simulink model "Turntable_Spawn"  (R2021a)
settings: Solver=ode4  StartTime=0.0  StopTime=inf  FixedStep=1/120  RelTol=1e-3  EnableMultiTasking=on
libraries: quarc_library x9, simulink x2
settings Model: SimulationMode=external  ExtModeTrigDuration=10000  Creator=MLevis  LastModifiedBy=swhitmell
settings SolverCC: AlgebraicLoopSolver=TrustRegion  PositivePriorityOrder=on
settings DataIOCC: ReturnWorkspaceOutputs=off
settings DebuggingCC: SFMachineParentedDataDiag=warning  ArithmeticOperatorsInVariantConditions=warning
settings HardwareCC: ProdBitPerPointer=32  ProdBitPerSizeT=32  ProdBitPerPtrDiffT=32  ProdLargestAtomicInteger=Long  ProdLargestAtomicFloat=Double  ProdWordSize=32  ProdHWDeviceType=ARM Compatible->ARM Cortex
settings SFSimCC: SimUseLocalCustomCode=off  CustomCodeUndefinedFunction=UseInterfaceOnly
settings RTWCC: Description=QUARC Linux Raspberry Pi 3 Target (QBot 2e) Using Toolchain  SystemTargetFile=quarc_linux_pi_3.tlc  TemplateMakefile=quarc_default_tmf  RTWUseLocalCustomCode=off  Toolchain=QUARC linux_pi_3 | gmake (64-bit Windows)  BuildConfiguration=Faster Runs
settings CodeAppCC: StateflowObjectComments=on
settings STFCustomTargetCC: TargetLangStandard=C99 (ISO)  ConcurrentExecutionCompliant=on  SystemTargetFile=quarc_linux_pi_3.tlc
settings GRTTargetCC: ParMdlRefBuildCompliant=off  CompOptLevelCompliant=off  CombineOutputUpdateFcns=off  MatFileLogging=off  CPPClassGenCompliant=off  GRTInterface=on  ExtMode=on  ExtModeMexFile=quarc_comm  ExtModeMexArgs='-w -d /tmp -uri %u'
settings ConfigComp: CovMetricSettings=dswe

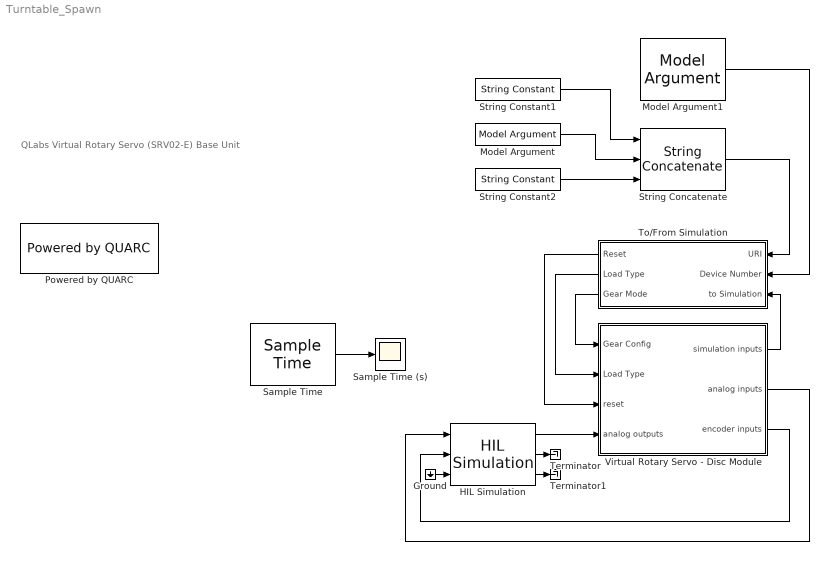
== system Turntable_Spawn ==
  note: QLabs Virtual Rotary Servo (SRV02-E)
      | Base Unit
  Ground : Ground
  HIL Simulation : quarc_library/Data Acquisition/Generic/Configuration/HIL Simulation  uri=tcpip://localhost:18940  board_type=q8_usb  board_id=0  sample_time=qc_get_step_size  active=on  num_clocks=1  num_interrupts=0  num_analog_inputs=8  num_analog_outputs=8  initial_analog=[]  num_digital_io=0  num_digital_inputs=8  num_digital_outputs=8  initial_digital=[]  num_encoder_inputs=8  num_pwm_outputs=8  initial_pwm=[]  other_inputs=[]  other_outputs=[]  initial_other=[]  integer_properties=[]  double_properties=[]  string_properties=[]
      settings: SourceProductName=QUARC Targets
  Model Argument : quarc_library/Sources/Signals/Model Argument  argument_name=hostname  has_value=on  data_type_mode=Specify via dialog  data_type=char  max_length=80  default_value=0  default_string=localhost  variable_size=off
      settings: AttributesFormatString=(-%<argument_name>)  SourceProductName=QUARC Targets
  Model Argument1 : quarc_library/Sources/Signals/Model Argument  argument_name=devicenum  has_value=on  data_type_mode=Specify via dialog  data_type=int32  max_length=80  default_value=0  variable_size=off
      settings: AttributesFormatString=(-%<argument_name>)  SourceProductName=QUARC Targets
  Powered by QUARC : quarc_library/Logos/Powered by QUARC
  Sample Time : quarc_library/Sources/Time/Sample Time  Priority=-99  sample_time=qc_get_step_size
  Sample Time (s) : Scope
  String Concatenate : quarc_library/Strings/String Concatenate  num_inputs=3  max_length=80  output_size=Inherit from input
      settings: SourceProductName=QUARC Targets
  String Constant1 : quarc_library/Strings/String Constant  string_value=tcpip://  evaluate_string=off  string_type=text  max_length=80  sample_time=inf  variable_size=off
      settings: AttributesFormatString="\"tcpip://\""  SourceProductName=QUARC Targets
  String Constant2 : quarc_library/Strings/String Constant  string_value=:18000?nagle='off'  evaluate_string=off  string_type=text  max_length=80  sample_time=inf  variable_size=off
      settings: AttributesFormatString="\":18000?nagle='off'\""  SourceProductName=QUARC Targets
  Terminator : Terminator
  Terminator1 : Terminator
  To/From Simulation : Subsystem
  Virtual Rotary Servo - Disc Module : Subsystem
  wires:
  To/From Simulation/2(Load Type) -> Virtual Rotary Servo - Disc Module/2(Load Type)
  Virtual Rotary Servo - Disc Module/3(encoder inputs) -> HIL Simulation/2
  Virtual Rotary Servo - Disc Module/2(analog inputs) -> HIL Simulation/1
  HIL Simulation/1 -> Virtual Rotary Servo - Disc Module/4(analog outputs)
  Sample Time/1 -> Sample Time (s)/1
  Virtual Rotary Servo - Disc Module/1(simulation inputs) -> To/From Simulation/3(to Simulation)
  To/From Simulation/1(Reset) -> Virtual Rotary Servo - Disc Module/3(reset)
  Ground/1 -> HIL Simulation/3
  HIL Simulation/2 -> Terminator/1
  HIL Simulation/3 -> Terminator1/1
  To/From Simulation/3(Gear Mode) -> Virtual Rotary Servo - Disc Module/1(Gear Config)
  Model Argument/1 -> String Concatenate/2
  String Constant2/1 -> String Concatenate/3
  String Constant1/1 -> String Concatenate/1
  String Concatenate/1 -> To/From Simulation/1(URI)
  Model Argument1/1 -> To/From Simulation/2(Device Number)

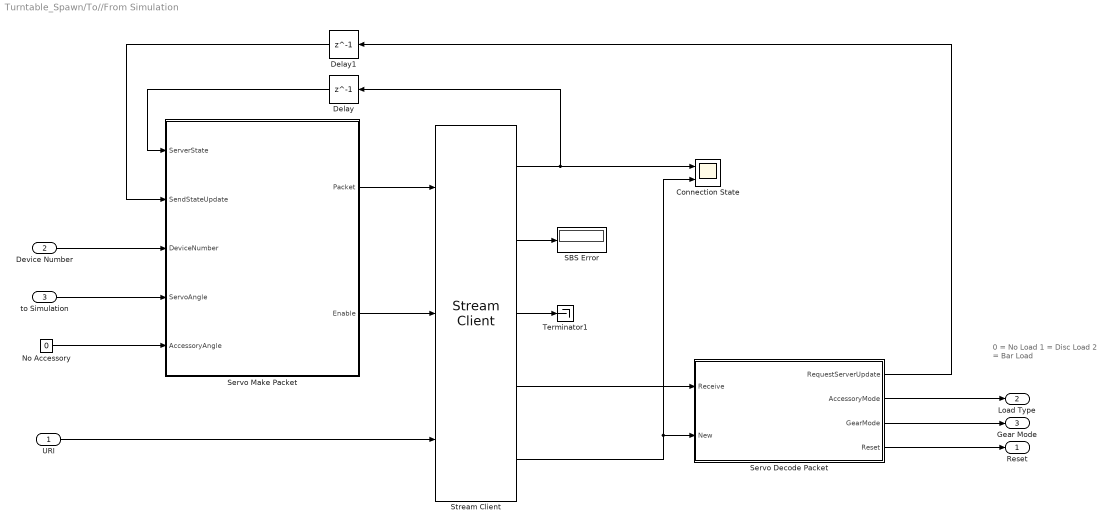
== system Turntable_Spawn/To//From Simulation ==
  note: 0 = No Load
      | 1 = Disc Load
      | 2 = Bar Load
  URI : Inport
  Device Number : Inport  Port=2
  to Simulation : Inport  Port=3
  "Connection State " : Scope  NumInputPorts=2
  Delay : Delay  DelayLength=1
  Delay1 : Delay  DelayLength=1
  No Accessory : Constant  Value=0
  SBS Error : Display
  Servo Decode Packet : MATLAB Function  TreatAsAtomicUnit=on
  Servo Make Packet : MATLAB Function  TreatAsAtomicUnit=on
  Stream Client : quarc_library/Communications/Basic/Stream Client  uri_source=External input port  uri=tcpip://remotehost:18000  apply_uri_to_all_configs=on  send_buffer_size=65537  receive_buffer_size=100000  byte_order=little endian (Intel - LSB first)  optimization=Minimum latency  send_options=Send all data  receive_options=Receive all data  default_value=[0]  sample_time=qc_get_step_size  active=on  implementation=Use blocking I/O in a separate thread  send_fifo_size=3  receive_fifo_size=3  send_priority=0  receive_priority=0  send_dimensions=on  receive_dimensions=on  max_dimensions=100000  data_type=uint8  type_expr=BusObject
  Terminator1 : Terminator
  Reset : Outport  VectorParamsAs1DForOutWhenUnconnected=off
  Load Type : Outport  Port=2  VectorParamsAs1DForOutWhenUnconnected=off
  Gear Mode : Outport  Port=3  VectorParamsAs1DForOutWhenUnconnected=off
  wires:
  Servo Decode Packet/2(AccessoryMode) -> Load Type/1
  Stream Client/2 -> SBS Error/1
  Servo Decode Packet/4(Reset) -> Reset/1
  Stream Client/3 -> Terminator1/1
  Stream Client/1 -> Delay/1, "Connection State "/1
  Servo Make Packet/2(Enable) -> Stream Client/2
  Servo Decode Packet/1(RequestServerUpdate) -> Delay1/1
  Stream Client/5 -> "Connection State "/2, Servo Decode Packet/2(New)
  Servo Make Packet/1(Packet) -> Stream Client/1
  Stream Client/4 -> Servo Decode Packet/1(Receive)
  No Accessory/1 -> Servo Make Packet/5(AccessoryAngle)
  to Simulation/1 -> Servo Make Packet/4(ServoAngle)
  Device Number/1 -> Servo Make Packet/3(DeviceNumber)
  Delay1/1 -> Servo Make Packet/2(SendStateUpdate)
  Delay/1 -> Servo Make Packet/1(ServerState)
  Servo Decode Packet/3(GearMode) -> Gear Mode/1
  URI/1 -> Stream Client/3

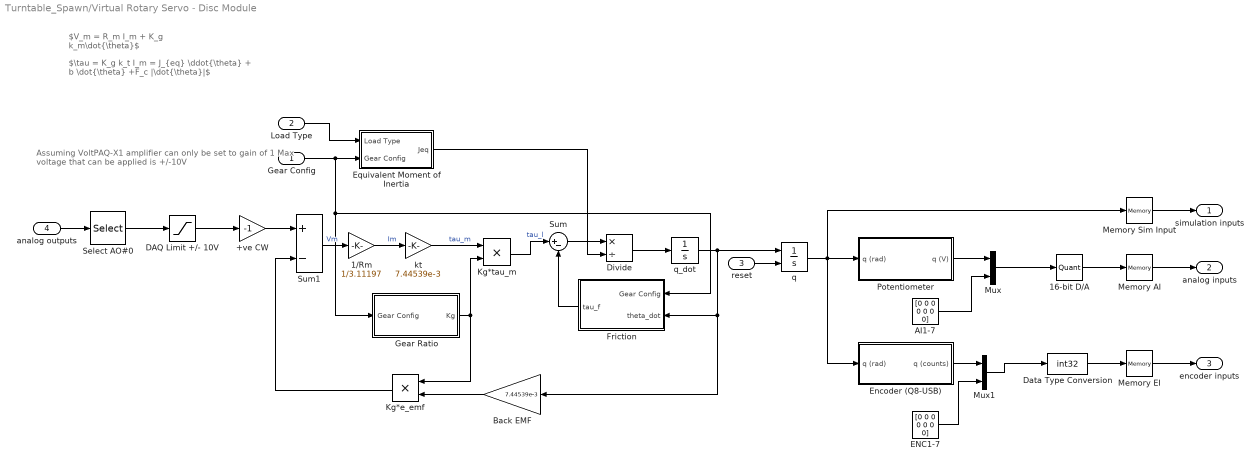
== system Turntable_Spawn/Virtual Rotary Servo - Disc Module ==
  note: $\tau = K_g k_t I_m = J_{eq} \ddot{\theta} + b \dot{\theta} +F_c |\dot{\theta}|$
  note: Assuming VoltPAQ-X1 amplifier can only be set to gain of 1
      | Max voltage that can be applied is +/-10V
  note: $V_m = R_m I_m + K_g k_m\dot{\theta}$
  Gear Config : Inport
  Load Type : Inport  Port=2
  reset : Inport  Port=3
  analog outputs : Inport  Port=4
  +ve CW : Gain  Gain=-1
  1/Rm : Gain  Gain=1/3.11197
  16-bit D/A : Quantizer  QuantizationInterval=1/2^16
  AI1-7 : Constant  Value=[0 0 0 0 0 0 0]
  Back EMF : Gain  Gain=7.44539e-3
  DAQ Limit +/- 10V : Saturate  UpperLimit=10  LowerLimit=-10
  Data Type Conversion : DataTypeConversion  OutDataTypeStr=int32
  Divide : Product  Inputs=*/
  ENC1-7 : Constant  Value=[0 0 0 0 0 0 0]
  Encoder (Q8-USB) : Subsystem
  Equivalent Moment of Inertia : Subsystem
  Friction : Subsystem
  Gear Ratio : Subsystem
  Kg*e_emf : Product
  Kg*tau_m : Product
  Memory AI : Memory  InheritSampleTime=on
  Memory EI : Memory  InheritSampleTime=on
  Memory Sim Input : Memory  InheritSampleTime=on
  Mux : Mux  Inputs=2
  Mux1 : Mux  Inputs=2
  Potentiometer : Subsystem
  Select AO#0 : Selector  InputPortWidth=8  IndexOptions=Index vector (dialog)  Indices=[1]  OutputSizes=1
  Sum : Sum  Inputs=|+-
  Sum1 : Sum  Inputs=+-
  kt : Gain  Gain=7.44539e-3
  q : Integrator  ExternalReset=either
  q_dot : Integrator
  simulation inputs : Outport  VectorParamsAs1DForOutWhenUnconnected=off
  analog inputs : Outport  Port=2  VectorParamsAs1DForOutWhenUnconnected=off
  encoder inputs : Outport  Port=3  VectorParamsAs1DForOutWhenUnconnected=off
  wires:
  kt/1 -> Kg*tau_m/1  "tau_m"
  Mux/1 -> 16-bit D/A/1
  Potentiometer/1(q (V)) -> Mux/1
  AI1-7/1 -> Mux/2
  Mux1/1 -> Data Type Conversion/1
  Encoder (Q8-USB)/1(q (counts)) -> Mux1/1
  ENC1-7/1 -> Mux1/2
  Equivalent Moment of Inertia/1(Jeq) -> Divide/2
  Divide/1 -> q_dot/1
  Sum/1 -> Divide/1
  Friction/1(tau_f) -> Sum/2
  Gear Ratio/1(Kg) -> Kg*e_emf/1, Kg*tau_m/2
  Back EMF/1 -> Kg*e_emf/2
  Gear Config/1 -> Equivalent Moment of Inertia/2(Gear Config), Friction/1(Gear Config), Gear Ratio/1(Gear Config)
  q/1 -> Memory Sim Input/1, Potentiometer/1(q (rad)), Encoder (Q8-USB)/1(q (rad))
  reset/1 -> q/2
  Load Type/1 -> Equivalent Moment of Inertia/1(Load Type)
  16-bit D/A/1 -> Memory AI/1
  +ve CW/1 -> Sum1/1
  Data Type Conversion/1 -> Memory EI/1
  analog outputs/1 -> Select AO#0/1
  Select AO#0/1 -> DAQ Limit +/- 10V/1
  Kg*tau_m/1 -> Sum/1  "tau_l"
  Kg*e_emf/1 -> Sum1/2
  q_dot/1 -> Friction/2(theta_dot), Back EMF/1, q/1
  Sum1/1 -> 1/Rm/1  "Vm"
  1/Rm/1 -> kt/1  "Im"
  DAQ Limit +/- 10V/1 -> +ve CW/1
  Memory AI/1 -> analog inputs/1
  Memory EI/1 -> encoder inputs/1
  Memory Sim Input/1 -> simulation inputs/1

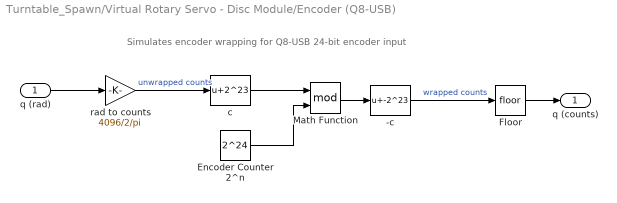
== system Turntable_Spawn/Virtual Rotary Servo - Disc Module/Encoder (Q8-USB) ==
  note: Simulates encoder wrapping for Q8-USB 24-bit encoder input
  q (rad) : Inport
  -c : Bias  Bias=-2^23
  Encoder Counter 2^n : Constant  Value=2^24
  Floor : Rounding
  Math Function : Math  Operator=mod  SignedPower=on  SaturateOnIntegerOverflow=on
  c : Bias  Bias=2^23
  rad to counts : Gain  Gain=4096/2/pi
  q (counts) : Outport  VectorParamsAs1DForOutWhenUnconnected=off
  wires:
  Floor/1 -> q (counts)/1
  -c/1 -> Floor/1  "wrapped counts"
  rad to counts/1 -> c/1  "unwrapped counts"
  Encoder Counter 2^n/1 -> Math Function/2
  c/1 -> Math Function/1
  q (rad)/1 -> rad to counts/1
  Math Function/1 -> -c/1

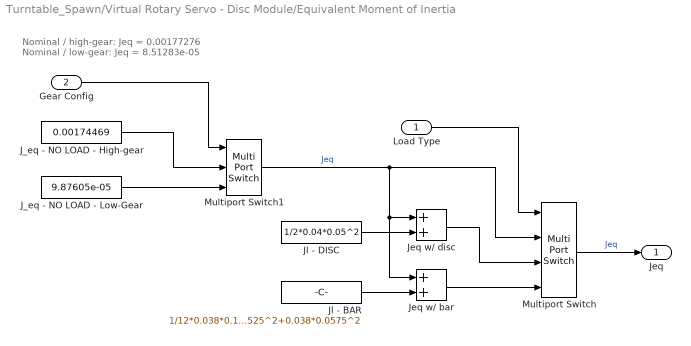
== system Turntable_Spawn/Virtual Rotary Servo - Disc Module/Equivalent Moment of Inertia ==
  note: Nominal / high-gear: Jeq = 0.00177276
      | Nominal / low-gear: Jeq = 8.51283e-05
  Load Type : Inport
  Gear Config : Inport  Port=2
  J_eq - NO LOAD - High-gear : Constant  Value=0.00174469
  J_eq - NO LOAD - Low-Gear : Constant  Value=9.87605e-05
  Jeq w/ bar : Sum
  Jeq w/ disc : Sum
  Jl - BAR : Constant  Value=1/12*0.038*0.1525^2+0.038*0.0575^2
  Jl - DISC : Constant  Value=1/2*0.04*0.05^2
  Multiport Switch : MultiPortSwitch  DataPortOrder=Zero-based contiguous  zeroidx=on
  Multiport Switch1 : MultiPortSwitch  DataPortOrder=Zero-based contiguous  Inputs=2  zeroidx=on
  Jeq : Outport  VectorParamsAs1DForOutWhenUnconnected=off
  wires:
  J_eq - NO LOAD - Low-Gear/1 -> Multiport Switch1/3
  J_eq - NO LOAD - High-gear/1 -> Multiport Switch1/2
  Multiport Switch/1 -> Jeq/1  "Jeq"
  Multiport Switch1/1 -> Multiport Switch/2, Jeq w/ disc/1, Jeq w/ bar/1  "Jeq"
  Gear Config/1 -> Multiport Switch1/1
  Jeq w/ disc/1 -> Multiport Switch/3
  Load Type/1 -> Multiport Switch/1
  Jeq w/ bar/1 -> Multiport Switch/4
  Jl - BAR/1 -> Jeq w/ bar/2
  Jl - DISC/1 -> Jeq w/ disc/2

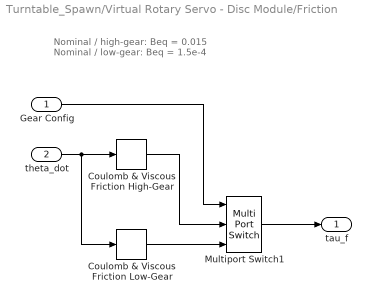
== system Turntable_Spawn/Virtual Rotary Servo - Disc Module/Friction ==
  note: Nominal / high-gear: Beq = 0.015
      | Nominal / low-gear: Beq = 1.5e-4
  Gear Config : Inport
  theta_dot : Inport  Port=2
  Coulomb & Viscous Friction High-Gear : simulink/Discontinuities/Coulomb & Viscous Friction  offset=0.030885  gain=0.0024798
  Coulomb & Viscous Friction Low-Gear : simulink/Discontinuities/Coulomb & Viscous Friction  offset=0.00502178  gain=1.19207e-04
  Multiport Switch1 : MultiPortSwitch  DataPortOrder=Zero-based contiguous  Inputs=2  zeroidx=on
  tau_f : Outport  VectorParamsAs1DForOutWhenUnconnected=off
  wires:
  Coulomb & Viscous Friction Low-Gear/1 -> Multiport Switch1/3
  theta_dot/1 -> Coulomb & Viscous Friction Low-Gear/1, Coulomb & Viscous Friction High-Gear/1
  Coulomb & Viscous Friction High-Gear/1 -> Multiport Switch1/2
  Gear Config/1 -> Multiport Switch1/1
  Multiport Switch1/1 -> tau_f/1

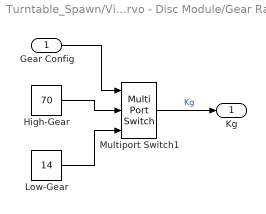
== system Turntable_Spawn/Virtual Rotary Servo - Disc Module/Gear Ratio ==
  Gear Config : Inport
  High-Gear : Constant  Value=70
  Low-Gear : Constant  Value=14
  Multiport Switch1 : MultiPortSwitch  DataPortOrder=Zero-based contiguous  Inputs=2  zeroidx=on
  Kg : Outport  VectorParamsAs1DForOutWhenUnconnected=off
  wires:
  Low-Gear/1 -> Multiport Switch1/3
  High-Gear/1 -> Multiport Switch1/2
  Gear Config/1 -> Multiport Switch1/1
  Multiport Switch1/1 -> Kg/1  "Kg"

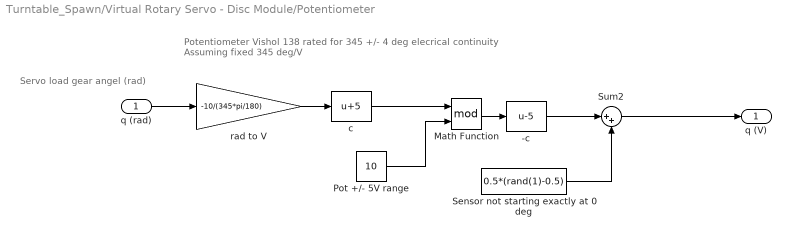
== system Turntable_Spawn/Virtual Rotary Servo - Disc Module/Potentiometer ==
  note: Potentiometer Vishol 138 rated for 345 +/- 4 deg elecrical continuity
      | Assuming fixed 345 deg/V
  note: Servo load gear angel (rad)
  q (rad) : Inport
  -c : Bias  Bias=-5
  Math Function : Math  Operator=mod  SignedPower=on  SaturateOnIntegerOverflow=on
  Pot +/- 5V range : Constant  Value=10
  Sensor not starting exactly at 0 deg : Constant  Value=0.5*(rand(1)-0.5)
  Sum2 : Sum  Inputs=|++
  c : Bias  Bias=5
  rad to V : Gain  Gain=-10/(345*pi/180)
  q (V) : Outport  VectorParamsAs1DForOutWhenUnconnected=off
  wires:
  Sum2/1 -> q (V)/1
  Math Function/1 -> -c/1
  c/1 -> Math Function/1
  rad to V/1 -> c/1
  Pot +/- 5V range/1 -> Math Function/2
  q (rad)/1 -> rad to V/1
  -c/1 -> Sum2/1
  Sensor not starting exactly at 0 deg/1 -> Sum2/2

== matlab function Turntable_Spawn/To//From Simulation/Servo Make Packet ==
  settings: updateMethod=DISCRETE  sampleTime=qc_get_step_size
  data: Packet output size=65537; ServerState input; SendStateUpdate input; Enable output; DeviceNumber input; ServoAngle input; AccessoryAngle input
function [Packet,Enable] = ServoMakePacket(ServerState, SendStateUpdate, DeviceNumber, ServoAngle, AccessoryAngle) 

% Be sure to set the maximum signal size of the variable size Packet port 
% in Simulink->Edit Data of the editor window.  Size should be 65537 or
% larger to ensure that the stream server generates a 4 byte packet size.

%% Setup
persistent LastServerState;

if isempty(LastServerState)
    LastServerState = uint8(0);
end

Enable = 0;
Packet = uint8([]);

%% On connection
if ((ServerState == 2) && (LastServerState ~= 2))
    Packet = ServoMakeCommandStateContainer(DeviceNumber, ServoAngle, AccessoryAngle); 
    Packet = [Packet; MakeModeRequestContainer(40, DeviceNumber)];
end

%% Send new State Container
% Previous state processed, send a new one
if (SendStateUpdate)
    Packet = ServoMakeCommandStateContainer(DeviceNumber, ServoAngle, AccessoryAngle); 
end

%% Transmit
% If we have data to send, enable the transmit
PacketLength = length(Packet);

if (PacketLength > 0)
    % Add magic byte.  This is just for error handling and isn't typically
    % required in simulink, but useful in lower-level languages like Python
    Packet = [uint8(123); Packet];
    
    Enable = 1; 
end


LastServerState = ServerState;

== matlab function Turntable_Spawn/To//From Simulation/Servo Decode Packet ==
  data: Receive input size=100000; RequestServerUpdate output; New input; AccessoryMode output; GearMode output; Reset output
function [RequestServerUpdate, AccessoryMode, GearMode, Reset] = ServoDecodePacket(Receive, New)

%% Setup

persistent iAccMode;
persistent iGearMode;

if isempty(iAccMode)
    iAccMode = uint8(0);
    iGearMode = uint8(0);
end

% Need to assign outputs here even though they are reassigned at the end
% since matlab can't determine the signal widths
AccessoryMode = uint8(0);
GearMode = uint8(0);
Reset = 0;
RequestServerUpdate = 0;

PacketSize = length(Receive);

% Packet > 0, new data, and magic number in first index
if ((PacketSize > 0) && (New == 1) && (Receive(1) == uint8(123)))
    
    %skip magic number
    Index = int32(2);
    
    while(Index <= PacketSize)
       
        %% Get container details
        ContainerSize = typecast(uint8(flip(Receive(Index:Index+3))), 'int32');
        DeviceID = typecast(uint8(flip(Receive(Index+4:Index+7))), 'int32');
        DeviceNum = typecast(uint8(flip(Receive(Index+8:Index+11))), 'int32');
        DeviceFunction = uint8(Receive(Index+12));
        PayloadStart = Index+13;
        PayloadEnd = Index+ContainerSize-1;
        
        %% Pass container to appropriate decoding function
        if (DeviceID == 40) %is this a SRV02 container?
            
            if (DeviceFunction == 11) %UE4 State Response
                RequestServerUpdate = 1;
            elseif (DeviceFunction == 13) %Mode change
                iAccMode = uint8(Receive(PayloadStart));
                iGearMode = uint8(Receive(PayloadStart + 1));
            end
        
        elseif (DeviceID == 1001) %Simulink notification
            if (DeviceFunction == 200) %Reset button
                Reset = 1;
            end
        end
        
        
        
        %% Process next container if any data is left.
        Index = Index+ContainerSize;
    end


end

AccessoryMode = iAccMode;
GearMode = iGearMode;
